simulink model "pcm"  (R2020a)
settings: Solver=VariableStepAuto  StartTime=0.0  StopTime=100  RelTol=1e-3
libraries: commutil2 x2, dspquant2 x2, commchan3 x1, dsparch4 x1, dspsigops x1
settings Model: Creator=Rohit  LastModifiedBy=Rohit

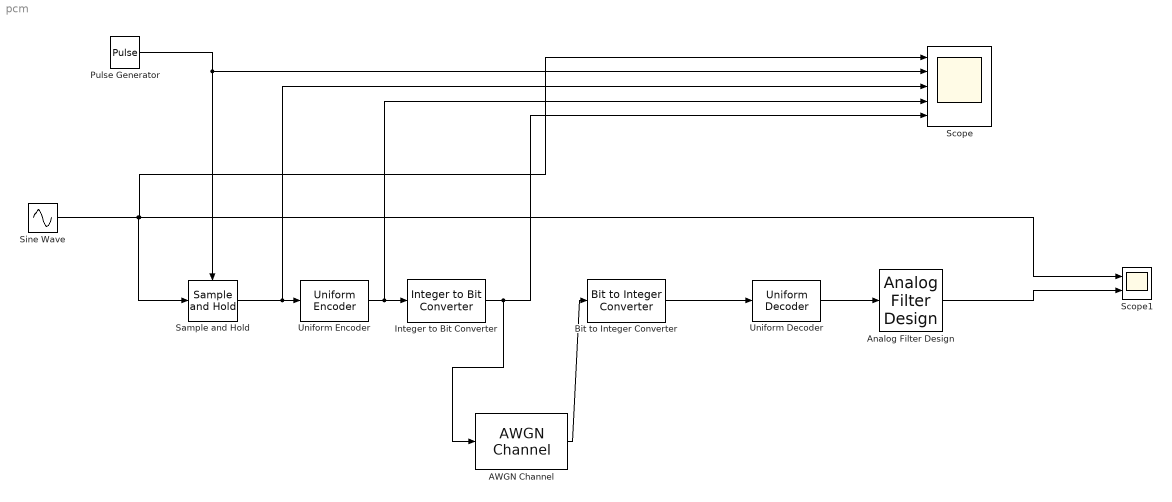
== system pcm ==
  AWGN Channel : commchan3/AWGN Channel  InputProcessing=Columns as channels (frame based)  seed=67  noiseMode="Signal to noise ratio  (Eb/No)"  EbNodB=10  EsNodB=10  SNRdB=10  bitsPerSym=1  Ps=1  Tsym=1  variance=1
  Analog Filter Design : dsparch4/Analog Filter Design  method=Butterworth  filttype=Lowpass  N=8  Wlo=3.5*pi  Whi=80  Rp=2  Rs=40
  Bit to Integer Converter : commutil2/Bit to Integer Converter  nbits=3  bitOrder=MSB first  signedOutputValues=Unsigned  outDtype=Inherit via internal rule  outDtypeSigned=Inherit via internal rule
  Integer to Bit Converter : commutil2/Integer to Bit Converter  nbits=3  signedInputValues=Unsigned  bitOrder=MSB first  outDtype=Inherit via internal rule
  Pulse Generator : DiscretePulseGenerator  PulseType=Time based  Period=0.1  PulseWidth=50
  Sample and Hold : dspsigops/Sample and Hold  trig=Rising edge  initCond=0  latchinput=off
  Scope : Scope  NumInputPorts=5
  Scope1 : Scope  NumInputPorts=2
  Sine Wave : Sin  Frequency=2*pi  SampleTime=0
  Uniform Decoder : dspquant2/Uniform Decoder  peak=1  bits=3  overflowMode=Saturate  otype=Double
      settings: SourceProductBaseCode=DS
  Uniform Encoder : dspquant2/Uniform Encoder  peak=1  bits=8  otype=Unsigned integer
  wires:
  Sine Wave/1 -> Sample and Hold/1, Scope/1, Scope1/1
  Sample and Hold/1 -> Scope/3, Uniform Encoder/1
  Uniform Encoder/1 -> Scope/4, Integer to Bit Converter/1
  Integer to Bit Converter/1 -> AWGN Channel/1, Scope/5
  Bit to Integer Converter/1 -> Uniform Decoder/1
  Uniform Decoder/1 -> Analog Filter Design/1
  Analog Filter Design/1 -> Scope1/2
  Pulse Generator/1 -> Scope/2, Sample and Hold/Trigger
  AWGN Channel/1 -> Bit to Integer Converter/1
